simulink model "Antenna_block_example"  (R2021b)
settings: Solver=VariableStepAuto  StartTime=0.0  StopTime=2e-4  RelTol=1e-3
PreLoadFcn:
  | R = 100;
  | FreqCarrier = 5e9;
  | lambdaCarrier = physconst('lightspeed')/FreqCarrier;
  | 
  | Gt = 7.9988; %[dBi]
  | Gr = Gt; %[dBi]
  | Zin_t =56.2947 - 1j*4.2629; %[Ohm]
  | Zin_r = Zin_t; %[Ohm]
undefined symbols (not defined in the file or in its folder): physconst, S
libraries: simrfV2elements x4, simrfV2util1 x4, rfBudgetAnalyzer_lib x2, simrfV2sources1 x1
settings Model: Creator=The MathWorks, Inc.  LastModifiedBy=The MathWorks, Inc.
settings SolverCC: AlgebraicLoopSolver=TrustRegion
settings DebuggingCC: SFMachineParentedDataDiag=warning

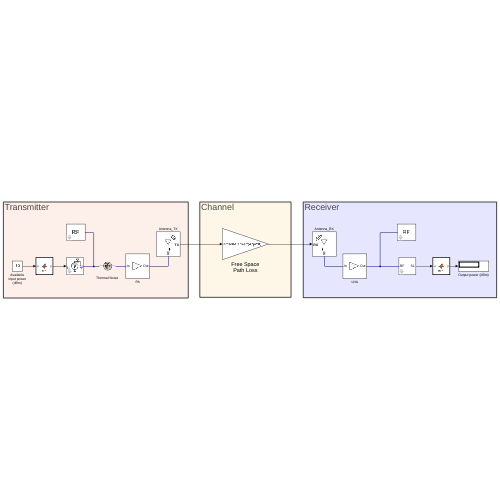
[thumbnail: Simulink's stored preview of the top-level diagram]
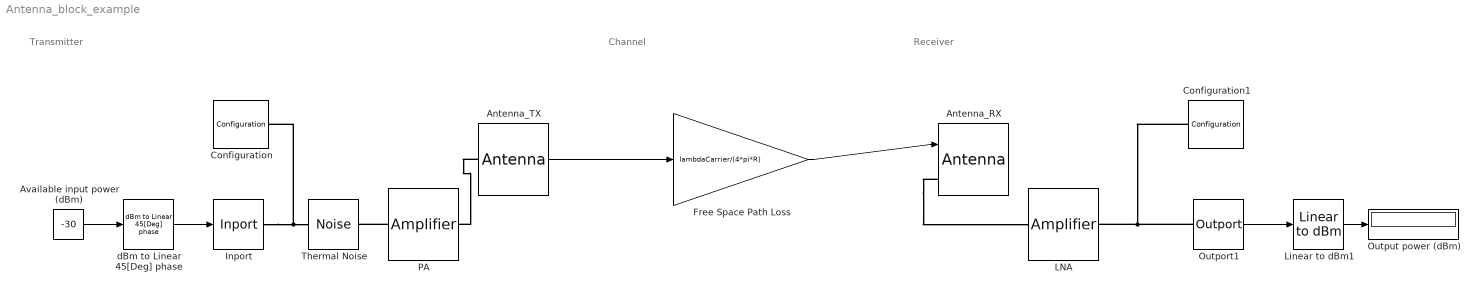
== system Antenna_block_example ==
  note: Channel
  note: Receiver
  note: Transmitter
  Antenna_RX : simrfV2elements/Antenna  AntennaSource=Isotropic radiator  PrevAppliedAntSource=Isotropic radiator  Gr=Gr dBi  Zin=Zin_r  AntennaObj=antObj  InputIncWave=on  OutputRadWave=off  CarrierFreqInc=FreqCarrier Hz  rArr=[0 -90] deg  CarrierFreqRad=FreqCarrier GHz  rDep=[0 0] deg  AddNoise=off  InternalGrounding=on  SparamRepresentationImp=Frequency domain  FitTolImp=-80  AutoImpulseLengthImp=off  ImpulseLengthImp=0 s
      settings: SourceProductBaseCode=RB
  Antenna_TX : simrfV2elements/Antenna  AntennaSource=Isotropic radiator  PrevAppliedAntSource=Isotropic radiator  Gr=Gt dBi  Zin=Zin_t  AntennaObj=antObj  InputIncWave=off  OutputRadWave=on  CarrierFreqInc=2.1 GHz  rArr=[180 0] deg  CarrierFreqRad=FreqCarrier Hz  rDep=[0 90] deg  AddNoise=off  InternalGrounding=on  SparamRepresentationImp=Frequency domain  FitTolImp=-80  AutoImpulseLengthImp=off  ImpulseLengthImp=0 s
      settings: SourceProductBaseCode=RB
  Available input power (dBm) : Constant  Value=-30
  Configuration : simrfV2util1/Configuration  AutoFreq=on  Tones=[5] GHz  Harmonics=[7]  NormalizeCarrierPower=on  SolverType=Auto  UseCCode=on  StepSize=(1/100000000)/8 s  AddNoise=off  defaultRNG=on  Seed=0  Temperature=290.0 K  SolverDelFlag=0  AbsTol=1e-6  RelTol=1e-3  MaxIter=10  ErrorEstimationType=2-norm over all variables  EnableInterpFilter=on  HiddenFIRfilterControllerParam=on  SmallSignalApprox=off  AllSimFreqs=on  SimFreqs=[] Hz  SimFreqsInternal=[]  SamplesPerFrame=1
      settings: SourceProductBaseCode=RB
  Configuration1 : simrfV2util1/Configuration  AutoFreq=on  Tones=[5] GHz  Harmonics=[7]  NormalizeCarrierPower=on  SolverType=Auto  UseCCode=on  StepSize=(1/100000000)/8 s  AddNoise=off  defaultRNG=on  Seed=0  Temperature=290.0 K  SolverDelFlag=0  AbsTol=1e-6  RelTol=1e-3  MaxIter=10  ErrorEstimationType=2-norm over all variables  EnableInterpFilter=on  HiddenFIRfilterControllerParam=on  SmallSignalApprox=off  AllSimFreqs=on  SimFreqs=[] Hz  SimFreqsInternal=[]  SamplesPerFrame=1
      settings: SourceProductBaseCode=RB
  Free Space Path Loss : Gain  Gain=lambdaCarrier/(4*pi*R)
  Inport : simrfV2util1/Inport  SimulinkInputSignalType=Power  CarrierFreq=FreqCarrier Hz  ZS=50  InternalGrounding=on
      settings: SourceProductBaseCode=RB
  LNA : simrfV2elements/Amplifier  classname=amplifier  DataSource=Data file  File=unitygain.s2p  Paramtype=S-parameters  Sparam=[0 0;1 0]  SparamFreq=1e9 Hz  SparamZ0=50  Residues=0  Poles=0  DF={0 0; 1 0}  Source_linear_gain=Available power gain  linear_gain=20 dB  Zin=Zin_r'  Zout=50  Source_Poly=Even and odd order  Poly_Coeffs=[0 1]  IPType=Output  IP2=inf dBm  IP3=inf dBm  P1dB=inf dBm  Psat=inf dBm  Gcomp=inf dBm  InternalGrounding=on  SourceFreq=Extracted from data source  PlotFreq=[1e9:1e6:3e9] Hz  PlotType=X-Y plane  YParam1=S(1,1)  YFormat1=Magnitude (decibels)  YParam2=None  YFormat2=Magnitude (decibels)  YOption=Linear  XOption=Linear  SparamRepresentation=Time domain (rationalfit)  FitTol=-40  FitOpt=Fit individually  MaxPoles=48  AutoImpulseLength=on  ImpulseLength=1e-10 s  MagModeling=off  AddNoise=on  NoiseType=Noise figure  NoiseDist=White  NF=0  MinNF=0  Gopt=0  RN=0  CarrierFreq=0 Hz  NoiseAutoImpulseLength=on  NoiseImpulseLength=1e-10 s  SpecifyOpFreq=off  OpFreq=0 Hz
      settings: SourceProductBaseCode=RB
  Linear to dBm1 : rfBudgetAnalyzer_lib/Linear to dBm  SystemSampleTime=-1  VariantActivationTime=update diagram  Latency=0  AutoFrameSizeCalculation=off
      settings: SourceProductBaseCode=RB
  Outport1 : simrfV2util1/Outport  SensorType=Power  OutputFormat=Complex Baseband  CarrierFreq=FreqCarrier Hz  ZL=50  InternalGrounding=on  StepSize=1e-6 s  AutoStep=on
      settings: SourceProductBaseCode=RB
  Output power (dBm) : Display
  PA : simrfV2elements/Amplifier  classname=amplifier  DataSource=Data file  File=unitygain.s2p  Paramtype=S-parameters  Sparam=[0 0;1 0]  SparamFreq=1e9 Hz  SparamZ0=50  Residues=0  Poles=0  DF={0 0; 1 0}  Source_linear_gain=Available power gain  linear_gain=35 dB  Zin=50  Zout=Zin_t'  Source_Poly=Even and odd order  Poly_Coeffs=[0 1]  IPType=Output  IP2=inf dBm  IP3=inf dBm  P1dB=inf dBm  Psat=inf dBm  Gcomp=inf dBm  InternalGrounding=on  SourceFreq=Extracted from data source  PlotFreq=[1e9:1e6:3e9] Hz  PlotType=X-Y plane  YParam1=S(1,1)  YFormat1=Magnitude (decibels)  YParam2=None  YFormat2=Magnitude (decibels)  YOption=Linear  XOption=Linear  SparamRepresentation=Time domain (rationalfit)  FitTol=-40  FitOpt=Fit individually  MaxPoles=48  AutoImpulseLength=on  ImpulseLength=1e-10 s  MagModeling=off  AddNoise=on  NoiseType=Noise figure  NoiseDist=White  NF=0  MinNF=0  Gopt=0  RN=0  CarrierFreq=0 Hz  NoiseAutoImpulseLength=on  NoiseImpulseLength=1e-10 s  SpecifyOpFreq=off  OpFreq=0 Hz
      settings: SourceProductBaseCode=RB
  Thermal Noise : simrfV2sources1/Noise  SimulinkInputSignalType=Ideal voltage  NoiseType=White  NoisePSD=4*physconst('Boltzmann')*290*50  CarrierFreq=0 Hz  AutoImpulseLength=on  ImpulseLength=1e-10 s  InternalGrounding=off
      settings: SourceProductBaseCode=RB
  dBm to Linear 45[Deg] phase : rfBudgetAnalyzer_lib/dBm to Linear 45[Deg] phase  SystemSampleTime=-1  VariantActivationTime=update diagram  Latency=0  AutoFrameSizeCalculation=off
      settings: SourceProductBaseCode=RB
  wires:
  Available input power (dBm)/1 -> dBm to Linear 45[Deg] phase/1
  dBm to Linear 45[Deg] phase/1 -> Inport/1
  Outport1/1 -> Linear to dBm1/1
  Linear to dBm1/1 -> Output power (dBm)/1
  Free Space Path Loss/1 -> Antenna_RX/1
  Antenna_TX/1 -> Free Space Path Loss/1
  connections:
  Configuration/LConn1 -- Inport/RConn1 -- Thermal Noise/RConn1
  PA/LConn1 -- Thermal Noise/LConn1
  Outport1/LConn1 -- Configuration1/LConn1 -- LNA/RConn1
  Antenna_RX/LConn1 -- LNA/LConn1
  Antenna_TX/LConn1 -- PA/RConn1
